simulink model "interpolation_nD_TestGen33"  (R2017b)
settings: Solver=FixedStepDiscrete  StartTime=0.0  StopTime=10.0  RelTol=1e-3
PreLoadFcn:
  |  LUTObj = Simulink.LookupTable;
  |  LUTObj.Table.Value = [101.281430812398 17.3423660349381;116.887406256746 42.6946846046885;71.404461183752 72.9554527021435];
  |  LUTObj.Table.DataType = 'auto';
  |  LUTObj.StructTypeInfo.Name = 'myLUTStruct';
  |  LUTObj.BreakpointsSpecification = 'Reference';
  |  LUTObj.Breakpoints{1} = 'myBpSet1';
  | myBpSet1 = Simulink.Breakpoint;
  | myBpSet1.Breakpoints.Value = [1 2 3];
  |  LUTObj.Breakpoints{2} = 'myBpSet2';
  | myBpSet2 = Simulink.Breakpoint;
  | myBpSet2.Breakpoints.Value = [1 2];
settings Model: Creator=ktrinh  LastModifiedBy=ktrinh
settings DebuggingCC: ParameterOverflowMsg=none

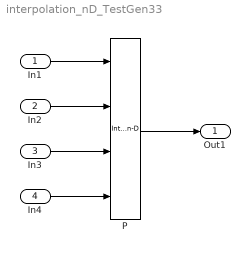
== system interpolation_nD_TestGen33 ==
  In1 : Inport  OutMin=0  OutMax=3  PortDimensions=3
  In2 : Inport  Port=2  OutMin=-0.5  OutMax=1.5
  In3 : Inport  Port=3  OutMin=0  OutMax=2
  In4 : Inport  Port=4  OutMin=-0.5  OutMax=1.5
  P : Interpolation_n-D  Table=[101.281430812398 17.3423660349381;116.887406256746 42.6946846046885;71.404461183752 72.9554527021435]  TableSpecification=Lookup table object  LookupTableObject=LUTObj  InterpMethod=Nearest  ExtrapMethod=Clip  ValidIndexMayReachLast=on  OutDataTypeStr=single  InternalRulePriority=Speed  RndMeth=Simplest  SaturateOnIntegerOverflow=on
  Out1 : Outport
  wires:
  In1/1 -> P/1
  In2/1 -> P/2
  In3/1 -> P/3
  In4/1 -> P/4
  P/1 -> Out1/1
